simulink library "halout"  (R2021b)
settings: Solver=VariableStepAuto  StartTime=0.0  StopTime=10.0  RelTol=1e-3
undefined symbols (not defined in the file): C_TASK_5MS_S, FALSE, KHAL_CAN1FD1APS3E2E_flg, KHAL_CAN1FD1APS3TxReq_flg, KHAL_CAN1FD1VCU2E2E_flg, KHAL_CAN1FD1VCU2TxReq_flg, KHAL_CAN1FD1VCU3E2E_flg, KHAL_CAN1FD1VCU3TxReq_flg, KHAL_CAN1TxReq_flg, KHAL_CAN1VMCFCM1E2E_flg, KHAL_CAN1VMCFCM1TxReq_flg, KHAL_CAN2TxReq_flg, KHAL_CAN3FD3VCU1toNIDECTxReq_flg, KHAL_CAN3FD3VCU1TxReq_flg, KHAL_CAN3FD3VCU2E2E_flg, KHAL_CAN3FD3VCU2toNIDECE2E_flg, KHAL_CAN3FD3VCU2toNIDECTxReq_flg, KHAL_CAN3FD3VCU2TxReq_flg, KHAL_CAN3TxReq_flg, KHAL_CAN4FD4CE1000E2E_flg, KHAL_CAN4FD4CE1000TxReq_flg, KHAL_CAN4TxReq_flg, KHAL_CAN5TxReq_flg, KHAL_CAN6FD6APS3E2E_flg, KHAL_CAN6FD6APS3TxReq_flg, KHAL_CAN6FD6VCU2E2E_flg, KHAL_CAN6FD6VCU2TxReq_flg, KHAL_CAN6TxReq_flg, ONE_INT, TRUE, ZERO_INT
libraries: FVT_lib x551, simulink x244
(part 23 of 26)

== system halout/HAL_OUT/CAN4/FD4_CE100_1_0x182/RrCoolanttemp ==
  RrCoolanttemp : Inport
  Data Type Conversion : DataTypeConversion  OutDataTypeStr=uint16  RndMeth=Round
  convert_out : FVT_lib/hal/convert_out  gain=1  offset=-40
  CAN4_Rr_Coolanttemp : Outport
  wires:
  Data Type Conversion/1 -> CAN4_Rr_Coolanttemp/1
  convert_out/1 -> Data Type Conversion/1
  RrCoolanttemp/1 -> convert_out/1

== system halout/HAL_OUT/CAN4/FD4_CE100_1_0x182/sigAirIntenZon1St ==
  sigAirIntenZon1St : Inport
  Data Type Conversion : DataTypeConversion  OutDataTypeStr=uint8  RndMeth=Round
  CAN4_sigAirIntenZon1St : Outport
  wires:
  Data Type Conversion/1 -> CAN4_sigAirIntenZon1St/1
  sigAirIntenZon1St/1 -> Data Type Conversion/1

== system halout/HAL_OUT/CAN4/FD4_CE100_1_0x182/sigAirIntenZon3St ==
  sigAirIntenZon3St : Inport
  Data Type Conversion : DataTypeConversion  OutDataTypeStr=uint8  RndMeth=Round
  CAN4_sigAirIntenZon3St : Outport
  wires:
  Data Type Conversion/1 -> CAN4_sigAirIntenZon3St/1
  sigAirIntenZon3St/1 -> Data Type Conversion/1

== system halout/HAL_OUT/CAN4/FD4_CE100_1_0x182/sigAmbAirT ==
  sigAmbAirT : Inport
  Data Type Conversion : DataTypeConversion  OutDataTypeStr=uint8  RndMeth=Round
  convert_out : FVT_lib/hal/convert_out  gain=0.5  offset=-40
  CAN4_sigAmbAirT : Outport
  wires:
  Data Type Conversion/1 -> CAN4_sigAmbAirT/1
  convert_out/1 -> Data Type Conversion/1
  sigAmbAirT/1 -> convert_out/1

== system halout/HAL_OUT/CAN4/FD4_CE100_1_0x182/sigCbnAirT ==
  sigCbnAirT : Inport
  Data Type Conversion : DataTypeConversion  OutDataTypeStr=uint8  RndMeth=Round
  convert_out : FVT_lib/hal/convert_out  gain=0.5  offset=-40
  CAN4_sigCbnAirT : Outport
  wires:
  Data Type Conversion/1 -> CAN4_sigCbnAirT/1
  convert_out/1 -> Data Type Conversion/1
  sigCbnAirT/1 -> convert_out/1

== system halout/HAL_OUT/CAN4/FD4_CE100_1_0x182/sigCbnPTCPwrAct ==
  sigCbnPTCPwrAct : Inport
  Data Type Conversion : DataTypeConversion  OutDataTypeStr=uint8  RndMeth=Round
  convert_out : FVT_lib/hal/convert_out  gain=50  offset=0
  CAN4_sigCbnPTCPwrAct : Outport
  wires:
  Data Type Conversion/1 -> CAN4_sigCbnPTCPwrAct/1
  convert_out/1 -> Data Type Conversion/1
  sigCbnPTCPwrAct/1 -> convert_out/1

== system halout/HAL_OUT/CAN4/FD4_CE100_1_0x182/sigCbnSolarLeft ==
  sigCbnSolarLeft : Inport
  Data Type Conversion : DataTypeConversion  OutDataTypeStr=uint8  RndMeth=Round
  convert_out : FVT_lib/hal/convert_out  gain=5  offset=0
  CAN4_sigCbnSolarLeft : Outport
  wires:
  Data Type Conversion/1 -> CAN4_sigCbnSolarLeft/1
  convert_out/1 -> Data Type Conversion/1
  sigCbnSolarLeft/1 -> convert_out/1

== system halout/HAL_OUT/CAN4/FD4_CE100_1_0x182/sigCbnSolarRight ==
  sigCbnSolarRight : Inport
  Data Type Conversion : DataTypeConversion  OutDataTypeStr=uint8  RndMeth=Round
  convert_out : FVT_lib/hal/convert_out  gain=5  offset=0
  CAN4_sigCbnSolarRight : Outport
  wires:
  Data Type Conversion/1 -> CAN4_sigCbnSolarRight/1
  convert_out/1 -> Data Type Conversion/1
  sigCbnSolarRight/1 -> convert_out/1

== system halout/HAL_OUT/CAN4/FD4_CE100_1_0x182/sigClmtCmprPwrAct ==
  sigClmtCmprPwrAct : Inport
  Data Type Conversion : DataTypeConversion  OutDataTypeStr=uint8  RndMeth=Round
  convert_out : FVT_lib/hal/convert_out  gain=50  offset=0
  CAN4_sigClmtCmprPwrAct : Outport
  wires:
  Data Type Conversion/1 -> CAN4_sigClmtCmprPwrAct/1
  convert_out/1 -> Data Type Conversion/1
  sigClmtCmprPwrAct/1 -> convert_out/1

== system halout/HAL_OUT/CAN4/FD4_CE100_1_0x182/sigClntTHvBattOut ==
  sigClntTHvBattOut : Inport
  Data Type Conversion : DataTypeConversion  OutDataTypeStr=uint8  RndMeth=Round
  convert_out : FVT_lib/hal/convert_out  gain=0.5  offset=-40
  CAN4_sigClntTHvBattOut : Outport
  wires:
  Data Type Conversion/1 -> CAN4_sigClntTHvBattOut/1
  convert_out/1 -> Data Type Conversion/1
  sigClntTHvBattOut/1 -> convert_out/1

== system halout/HAL_OUT/CAN4/FD4_CE100_1_0x182/sigDfrstSt ==
  sigDfrstSt : Inport
  Data Type Conversion : DataTypeConversion  OutDataTypeStr=uint8  RndMeth=Round
  CAN4_sigDfrstSt : Outport
  wires:
  Data Type Conversion/1 -> CAN4_sigDfrstSt/1
  sigDfrstSt/1 -> Data Type Conversion/1

== system halout/HAL_OUT/CAN4/FD4_CE100_1_0x182/sigHvacSt ==
  sigHvacSt : Inport
  Data Type Conversion : DataTypeConversion  OutDataTypeStr=uint8  RndMeth=Round
  CAN4_sigHvacSt : Outport
  wires:
  Data Type Conversion/1 -> CAN4_sigHvacSt/1
  sigHvacSt/1 -> Data Type Conversion/1

== system halout/HAL_OUT/CAN4/FD4_CE100_1_0x182/sigRecircSt ==
  sigRecircSt : Inport
  Data Type Conversion : DataTypeConversion  OutDataTypeStr=uint8  RndMeth=Round
  CAN4_sigRecircSt : Outport
  wires:
  Data Type Conversion/1 -> CAN4_sigRecircSt/1
  sigRecircSt/1 -> Data Type Conversion/1

== system halout/HAL_OUT/CAN4/FD4_CE100_1_0x182/sigSetTempZon1St ==
  sigSetTempZon1St : Inport
  Data Type Conversion : DataTypeConversion  OutDataTypeStr=uint8  RndMeth=Round
  convert_out : FVT_lib/hal/convert_out  gain=0.5  offset=17
  CAN4_sigSetTempZon1St : Outport
  wires:
  Data Type Conversion/1 -> CAN4_sigSetTempZon1St/1
  convert_out/1 -> Data Type Conversion/1
  sigSetTempZon1St/1 -> convert_out/1

== system halout/HAL_OUT/CAN4/FD4_CE100_1_0x182/sigSetTempZon2St ==
  sigSetTempZon2St : Inport
  Data Type Conversion : DataTypeConversion  OutDataTypeStr=uint8  RndMeth=Round
  convert_out : FVT_lib/hal/convert_out  gain=0.5  offset=17
  CAN4_sigSetTempZon2St : Outport
  wires:
  Data Type Conversion/1 -> CAN4_sigSetTempZon2St/1
  convert_out/1 -> Data Type Conversion/1
  sigSetTempZon2St/1 -> convert_out/1

== system halout/HAL_OUT/CAN4/FD4_CE100_1_0x182/sigSetTempZon3St ==
  sigSetTempZon3St : Inport
  Data Type Conversion : DataTypeConversion  OutDataTypeStr=uint8  RndMeth=Round
  convert_out : FVT_lib/hal/convert_out  gain=0.5  offset=17
  CAN4_sigSetTempZon3St : Outport
  wires:
  Data Type Conversion/1 -> CAN4_sigSetTempZon3St/1
  convert_out/1 -> Data Type Conversion/1
  sigSetTempZon3St/1 -> convert_out/1

== system halout/HAL_OUT/CAN4/FD4_CE100_1_0x182/sigWindDirZon1St ==
  sigWindDirZon1St : Inport
  Data Type Conversion : DataTypeConversion  OutDataTypeStr=uint8  RndMeth=Round
  CAN4_sigWindDirZon1St : Outport
  wires:
  Data Type Conversion/1 -> CAN4_sigWindDirZon1St/1
  sigWindDirZon1St/1 -> Data Type Conversion/1

== system halout/HAL_OUT/CAN4/FD4_CE100_1_0x182/sigWindDirZon3St ==
  sigWindDirZon3St : Inport
  Data Type Conversion : DataTypeConversion  OutDataTypeStr=uint8  RndMeth=Round
  CAN4_sigWindDirZon3St : Outport
  wires:
  Data Type Conversion/1 -> CAN4_sigWindDirZon3St/1
  sigWindDirZon3St/1 -> Data Type Conversion/1

== system halout/HAL_OUT/CAN4/FD4_CE200_0_0x217/AmbLightBreath1 ==
  AmbLightBreath1 : Inport
  Data Type Conversion : DataTypeConversion  OutDataTypeStr=uint8  RndMeth=Round
  CAN4_AmbLightBreath1 : Outport
  wires:
  Data Type Conversion/1 -> CAN4_AmbLightBreath1/1
  AmbLightBreath1/1 -> Data Type Conversion/1

== system halout/HAL_OUT/CAN4/FD4_CE200_0_0x217/AmbLightBreath2 ==
  AmbLightBreath2 : Inport
  Data Type Conversion : DataTypeConversion  OutDataTypeStr=uint8  RndMeth=Round
  CAN4_AmbLightBreath2 : Outport
  wires:
  Data Type Conversion/1 -> CAN4_AmbLightBreath2/1
  AmbLightBreath2/1 -> Data Type Conversion/1

== system halout/HAL_OUT/CAN4/FD4_CE200_0_0x217/AmbLightBreath3 ==
  AmbLightBreath3 : Inport
  Data Type Conversion : DataTypeConversion  OutDataTypeStr=uint8  RndMeth=Round
  CAN4_AmbLightBreath3 : Outport
  wires:
  Data Type Conversion/1 -> CAN4_AmbLightBreath3/1
  AmbLightBreath3/1 -> Data Type Conversion/1

== system halout/HAL_OUT/CAN4/FD4_CE200_0_0x217/AmbLightBreath4 ==
  AmbLightBreath4 : Inport
  Data Type Conversion : DataTypeConversion  OutDataTypeStr=uint8  RndMeth=Round
  CAN4_AmbLightBreath4 : Outport
  wires:
  Data Type Conversion/1 -> CAN4_AmbLightBreath4/1
  AmbLightBreath4/1 -> Data Type Conversion/1

== system halout/HAL_OUT/CAN4/FD4_CE200_0_0x217/AmbLightBreath5 ==
  AmbLightBreath5 : Inport
  Data Type Conversion : DataTypeConversion  OutDataTypeStr=uint8  RndMeth=Round
  CAN4_AmbLightBreath5 : Outport
  wires:
  Data Type Conversion/1 -> CAN4_AmbLightBreath5/1
  AmbLightBreath5/1 -> Data Type Conversion/1

== system halout/HAL_OUT/CAN4/FD4_CE200_0_0x217/AmbLightBreath6 ==
  AmbLightBreath6 : Inport
  Data Type Conversion : DataTypeConversion  OutDataTypeStr=uint8  RndMeth=Round
  CAN4_AmbLightBreath6 : Outport
  wires:
  Data Type Conversion/1 -> CAN4_AmbLightBreath6/1
  AmbLightBreath6/1 -> Data Type Conversion/1

== system halout/HAL_OUT/CAN4/FD4_CE200_0_0x217/AmbLightBrightness1 ==
  AmbLightBrightness1 : Inport
  Data Type Conversion : DataTypeConversion  OutDataTypeStr=uint8  RndMeth=Round
  CAN4_AmbLightBrightness1 : Outport
  wires:
  Data Type Conversion/1 -> CAN4_AmbLightBrightness1/1
  AmbLightBrightness1/1 -> Data Type Conversion/1

== system halout/HAL_OUT/CAN4/FD4_CE200_0_0x217/AmbLightBrightness2 ==
  AmbLightBrightness2 : Inport
  Data Type Conversion : DataTypeConversion  OutDataTypeStr=uint8  RndMeth=Round
  CAN4_AmbLightBrightness2 : Outport
  wires:
  Data Type Conversion/1 -> CAN4_AmbLightBrightness2/1
  AmbLightBrightness2/1 -> Data Type Conversion/1

== system halout/HAL_OUT/CAN4/FD4_CE200_0_0x217/AmbLightBrightness3 ==
  AmbLightBrightness3 : Inport
  Data Type Conversion : DataTypeConversion  OutDataTypeStr=uint8  RndMeth=Round
  CAN4_AmbLightBrightness3 : Outport
  wires:
  Data Type Conversion/1 -> CAN4_AmbLightBrightness3/1
  AmbLightBrightness3/1 -> Data Type Conversion/1

== system halout/HAL_OUT/CAN4/FD4_CE200_0_0x217/AmbLightBrightness4 ==
  AmbLightBrightness4 : Inport
  Data Type Conversion : DataTypeConversion  OutDataTypeStr=uint8  RndMeth=Round
  CAN4_AmbLightBrightness4 : Outport
  wires:
  Data Type Conversion/1 -> CAN4_AmbLightBrightness4/1
  AmbLightBrightness4/1 -> Data Type Conversion/1

== system halout/HAL_OUT/CAN4/FD4_CE200_0_0x217/AmbLightBrightness5 ==
  AmbLightBrightness5 : Inport
  Data Type Conversion : DataTypeConversion  OutDataTypeStr=uint8  RndMeth=Round
  CAN4_AmbLightBrightness5 : Outport
  wires:
  Data Type Conversion/1 -> CAN4_AmbLightBrightness5/1
  AmbLightBrightness5/1 -> Data Type Conversion/1

== system halout/HAL_OUT/CAN4/FD4_CE200_0_0x217/AmbLightBrightness6 ==
  AmbLightBrightness6 : Inport
  Data Type Conversion : DataTypeConversion  OutDataTypeStr=uint8  RndMeth=Round
  CAN4_AmbLightBrightness6 : Outport
  wires:
  Data Type Conversion/1 -> CAN4_AmbLightBrightness6/1
  AmbLightBrightness6/1 -> Data Type Conversion/1

== system halout/HAL_OUT/CAN4/FD4_CE200_0_0x217/AmbLightColor1 ==
  AmbLightColor1 : Inport
  Data Type Conversion : DataTypeConversion  OutDataTypeStr=uint8  RndMeth=Round
  CAN4_AmbLightColor1 : Outport
  wires:
  Data Type Conversion/1 -> CAN4_AmbLightColor1/1
  AmbLightColor1/1 -> Data Type Conversion/1

== system halout/HAL_OUT/CAN4/FD4_CE200_0_0x217/AmbLightColor2 ==
  AmbLightColor2 : Inport
  Data Type Conversion : DataTypeConversion  OutDataTypeStr=uint8  RndMeth=Round
  CAN4_AmbLightColor2 : Outport
  wires:
  Data Type Conversion/1 -> CAN4_AmbLightColor2/1
  AmbLightColor2/1 -> Data Type Conversion/1

== system halout/HAL_OUT/CAN4/FD4_CE200_0_0x217/AmbLightColor3 ==
  AmbLightColor3 : Inport
  Data Type Conversion : DataTypeConversion  OutDataTypeStr=uint8  RndMeth=Round
  CAN4_AmbLightColor3 : Outport
  wires:
  Data Type Conversion/1 -> CAN4_AmbLightColor3/1
  AmbLightColor3/1 -> Data Type Conversion/1

== system halout/HAL_OUT/CAN4/FD4_CE200_0_0x217/AmbLightColor4 ==
  AmbLightColor4 : Inport
  Data Type Conversion : DataTypeConversion  OutDataTypeStr=uint8  RndMeth=Round
  CAN4_AmbLightColor4 : Outport
  wires:
  Data Type Conversion/1 -> CAN4_AmbLightColor4/1
  AmbLightColor4/1 -> Data Type Conversion/1

== system halout/HAL_OUT/CAN4/FD4_CE200_0_0x217/AmbLightColor5 ==
  AmbLightColor5 : Inport
  Data Type Conversion : DataTypeConversion  OutDataTypeStr=uint8  RndMeth=Round
  CAN4_AmbLightColor5 : Outport
  wires:
  Data Type Conversion/1 -> CAN4_AmbLightColor5/1
  AmbLightColor5/1 -> Data Type Conversion/1

== system halout/HAL_OUT/CAN4/FD4_CE200_0_0x217/AmbLightColor6 ==
  AmbLightColor6 : Inport
  Data Type Conversion : DataTypeConversion  OutDataTypeStr=uint8  RndMeth=Round
  CAN4_AmbLightColor6 : Outport
  wires:
  Data Type Conversion/1 -> CAN4_AmbLightColor6/1
  AmbLightColor6/1 -> Data Type Conversion/1

== system halout/HAL_OUT/CAN4/FD4_CE200_0_0x217/BCMBuzzerReq ==
  BCMBuzzerReq : Inport
  Data Type Conversion : DataTypeConversion  OutDataTypeStr=uint8  RndMeth=Round
  CAN4_BCM_Buzzer_Req : Outport
  wires:
  Data Type Conversion/1 -> CAN4_BCM_Buzzer_Req/1
  BCMBuzzerReq/1 -> Data Type Conversion/1

== system halout/HAL_OUT/CAN4/FD4_CE200_0_0x217/FDCBCMATCtrlCmd ==
  FDCBCMATCtrlCmd : Inport
  Data Type Conversion : DataTypeConversion  OutDataTypeStr=uint8  RndMeth=Round
  CAN4_FDC_BCM_ATCtrl_Cmd : Outport
  wires:
  Data Type Conversion/1 -> CAN4_FDC_BCM_ATCtrl_Cmd/1
  FDCBCMATCtrlCmd/1 -> Data Type Conversion/1

== system halout/HAL_OUT/CAN4/FD4_CE200_0_0x217/FDCBCMDSEATentryfsetSta ==
  FDCBCMDSEATentryfsetSta : Inport
  Data Type Conversion : DataTypeConversion  OutDataTypeStr=uint8  RndMeth=Round
  CAN4_FDC_BCM_DSEATentryfset_Sta : Outport
  wires:
  Data Type Conversion/1 -> CAN4_FDC_BCM_DSEATentryfset_Sta/1
  FDCBCMDSEATentryfsetSta/1 -> Data Type Conversion/1

== system halout/HAL_OUT/CAN4/FD4_CE200_0_0x217/FDCBCMDimSw ==
  FDCBCMDimSw : Inport
  Data Type Conversion : DataTypeConversion  OutDataTypeStr=uint8  RndMeth=Round
  CAN4_FDC_BCM_DimSw : Outport
  wires:
  Data Type Conversion/1 -> CAN4_FDC_BCM_DimSw/1
  FDCBCMDimSw/1 -> Data Type Conversion/1

== system halout/HAL_OUT/CAN4/FD4_CE200_0_0x217/FDCBCMDrHandleLampCmd ==
  FDCBCMDrHandleLampCmd : Inport
  Data Type Conversion : DataTypeConversion  OutDataTypeStr=uint8  RndMeth=Round
  CAN4_FDC_BCM_DrHandleLamp_Cmd : Outport
  wires:
  Data Type Conversion/1 -> CAN4_FDC_BCM_DrHandleLamp_Cmd/1
  FDCBCMDrHandleLampCmd/1 -> Data Type Conversion/1

== system halout/HAL_OUT/CAN4/FD4_CE200_0_0x217/FDCBCMDrRWdwReqAPSta ==
  FDCBCMDrRWdwReqAPSta : Inport
  Data Type Conversion : DataTypeConversion  OutDataTypeStr=uint8  RndMeth=Round
  CAN4_FDC_BCM_DrRWdwReqAP_Sta : Outport
  wires:
  Data Type Conversion/1 -> CAN4_FDC_BCM_DrRWdwReqAP_Sta/1
  FDCBCMDrRWdwReqAPSta/1 -> Data Type Conversion/1

== system halout/HAL_OUT/CAN4/FD4_CE200_0_0x217/FDCBCMDrvWdwReqAPSta ==
  FDCBCMDrvWdwReqAPSta : Inport
  Data Type Conversion : DataTypeConversion  OutDataTypeStr=uint8  RndMeth=Round
  CAN4_FDC_BCM_DrvWdwReqAP_Sta : Outport
  wires:
  Data Type Conversion/1 -> CAN4_FDC_BCM_DrvWdwReqAP_Sta/1
  FDCBCMDrvWdwReqAPSta/1 -> Data Type Conversion/1

== system halout/HAL_OUT/CAN4/FD4_CE200_0_0x217/FDCBCMFWasSwSta ==
  FDCBCMFWasSwSta : Inport
  Data Type Conversion : DataTypeConversion  OutDataTypeStr=uint8  RndMeth=Round
  CAN4_FDC_BCM_FWasSw_Sta : Outport
  wires:
  Data Type Conversion/1 -> CAN4_FDC_BCM_FWasSw_Sta/1
  FDCBCMFWasSwSta/1 -> Data Type Conversion/1

== system halout/HAL_OUT/CAN4/FD4_CE200_0_0x217/FDCBCMFWipSwSta ==
  FDCBCMFWipSwSta : Inport
  Data Type Conversion : DataTypeConversion  OutDataTypeStr=uint8  RndMeth=Round
  CAN4_FDC_BCM_FWipSw_Sta : Outport
  wires:
  Data Type Conversion/1 -> CAN4_FDC_BCM_FWipSw_Sta/1
  FDCBCMFWipSwSta/1 -> Data Type Conversion/1

== system halout/HAL_OUT/CAN4/FD4_CE200_0_0x217/FDCBCMHBeamADBCmd ==
  FDCBCMHBeamADBCmd : Inport
  Data Type Conversion : DataTypeConversion  OutDataTypeStr=uint8  RndMeth=Round
  CAN4_FDC_BCM_HBeamADB_Cmd : Outport
  wires:
  Data Type Conversion/1 -> CAN4_FDC_BCM_HBeamADB_Cmd/1
  FDCBCMHBeamADBCmd/1 -> Data Type Conversion/1

== system halout/HAL_OUT/CAN4/FD4_CE200_0_0x217/FDCBCMHandleControlCmd ==
  FDCBCMHandleControlCmd : Inport
  Data Type Conversion : DataTypeConversion  OutDataTypeStr=uint8  RndMeth=Round
  CAN4_FDC_BCM_HandleControl_Cmd : Outport
  wires:
  Data Type Conversion/1 -> CAN4_FDC_BCM_HandleControl_Cmd/1
  FDCBCMHandleControlCmd/1 -> Data Type Conversion/1

== system halout/HAL_OUT/CAN4/FD4_CE200_0_0x217/FDCBCMHazardINDCmd ==
  FDCBCMHazardINDCmd : Inport
  Data Type Conversion : DataTypeConversion  OutDataTypeStr=uint8  RndMeth=Round
  CAN4_FDC_BCM_HazardIND_Cmd : Outport
  wires:
  Data Type Conversion/1 -> CAN4_FDC_BCM_HazardIND_Cmd/1
  FDCBCMHazardINDCmd/1 -> Data Type Conversion/1

== system halout/HAL_OUT/CAN4/FD4_CE200_0_0x217/FDCBCMHoodRelCmd ==
  FDCBCMHoodRelCmd : Inport
  Data Type Conversion : DataTypeConversion  OutDataTypeStr=uint8  RndMeth=Round
  CAN4_FDC_BCM_HoodRel_Cmd : Outport
  wires:
  Data Type Conversion/1 -> CAN4_FDC_BCM_HoodRel_Cmd/1
  FDCBCMHoodRelCmd/1 -> Data Type Conversion/1

== system halout/HAL_OUT/CAN4/FD4_CE200_0_0x217/FDCBCMLPSDCtrlCmd ==
  FDCBCMLPSDCtrlCmd : Inport
  Data Type Conversion : DataTypeConversion  OutDataTypeStr=uint8  RndMeth=Round
  CAN4_FDC_BCM_LPSDCtrl_Cmd : Outport
  wires:
  Data Type Conversion/1 -> CAN4_FDC_BCM_LPSDCtrl_Cmd/1
  FDCBCMLPSDCtrlCmd/1 -> Data Type Conversion/1

== system halout/HAL_OUT/CAN4/FD4_CE200_0_0x217/FDCBCMLockAlarmCmd ==
  FDCBCMLockAlarmCmd : Inport
  Data Type Conversion : DataTypeConversion  OutDataTypeStr=uint8  RndMeth=Round
  CAN4_FDC_BCM_LockAlarm_Cmd : Outport
  wires:
  Data Type Conversion/1 -> CAN4_FDC_BCM_LockAlarm_Cmd/1
  FDCBCMLockAlarmCmd/1 -> Data Type Conversion/1

== system halout/HAL_OUT/CAN4/FD4_CE200_0_0x217/FDCBCMOtHandleLampCmd ==
  FDCBCMOtHandleLampCmd : Inport
  Data Type Conversion : DataTypeConversion  OutDataTypeStr=uint8  RndMeth=Round
  CAN4_FDC_BCM_OtHandleLamp_Cmd : Outport
  wires:
  Data Type Conversion/1 -> CAN4_FDC_BCM_OtHandleLamp_Cmd/1
  FDCBCMOtHandleLampCmd/1 -> Data Type Conversion/1

== system halout/HAL_OUT/CAN4/FD4_CE200_0_0x217/FDCBCMOutModeCmd ==
  FDCBCMOutModeCmd : Inport
  Data Type Conversion : DataTypeConversion  OutDataTypeStr=uint8  RndMeth=Round
  CAN4_FDC_BCM_OutMode_Cmd : Outport
  wires:
  Data Type Conversion/1 -> CAN4_FDC_BCM_OutMode_Cmd/1
  FDCBCMOutModeCmd/1 -> Data Type Conversion/1

== system halout/HAL_OUT/CAN4/FD4_CE200_0_0x217/FDCBCMPTGOpenHeightSta ==
  FDCBCMPTGOpenHeightSta : Inport
  Data Type Conversion : DataTypeConversion  OutDataTypeStr=uint8  RndMeth=Round
  CAN4_FDC_BCM_PTGOpenHeight_Sta : Outport
  wires:
  Data Type Conversion/1 -> CAN4_FDC_BCM_PTGOpenHeight_Sta/1
  FDCBCMPTGOpenHeightSta/1 -> Data Type Conversion/1

== system halout/HAL_OUT/CAN4/FD4_CE200_0_0x217/FDCBCMPasWdwReqAPSta ==
  FDCBCMPasWdwReqAPSta : Inport
  Data Type Conversion : DataTypeConversion  OutDataTypeStr=uint8  RndMeth=Round
  CAN4_FDC_BCM_PasWdwReqAP_Sta : Outport
  wires:
  Data Type Conversion/1 -> CAN4_FDC_BCM_PasWdwReqAP_Sta/1
  FDCBCMPasWdwReqAPSta/1 -> Data Type Conversion/1

== system halout/HAL_OUT/CAN4/FD4_CE200_0_0x217/FDCBCMPassSWSta ==
  FDCBCMPassSWSta : Inport
  Data Type Conversion : DataTypeConversion  OutDataTypeStr=uint8  RndMeth=Round
  CAN4_FDC_BCM_PassSW_Sta : Outport
  wires:
  Data Type Conversion/1 -> CAN4_FDC_BCM_PassSW_Sta/1
  FDCBCMPassSWSta/1 -> Data Type Conversion/1

== system halout/HAL_OUT/CAN4/FD4_CE200_0_0x217/FDCBCMPsRWdwReqAPSta ==
  FDCBCMPsRWdwReqAPSta : Inport
  Data Type Conversion : DataTypeConversion  OutDataTypeStr=uint8  RndMeth=Round
  CAN4_FDC_BCM_PsRWdwReqAP_Sta : Outport
  wires:
  Data Type Conversion/1 -> CAN4_FDC_BCM_PsRWdwReqAP_Sta/1
  FDCBCMPsRWdwReqAPSta/1 -> Data Type Conversion/1

== system halout/HAL_OUT/CAN4/FD4_CE200_0_0x217/FDCBCMRPSDCtrlCmd ==
  FDCBCMRPSDCtrlCmd : Inport
  Data Type Conversion : DataTypeConversion  OutDataTypeStr=uint8  RndMeth=Round
  CAN4_FDC_BCM_RPSDCtrl_Cmd : Outport
  wires:
  Data Type Conversion/1 -> CAN4_FDC_BCM_RPSDCtrl_Cmd/1
  FDCBCMRPSDCtrlCmd/1 -> Data Type Conversion/1

== system halout/HAL_OUT/CAN4/FD4_CE200_0_0x217/FDCBCMSettingUpdateReqCmd ==
  FDCBCMSettingUpdateReqCmd : Inport
  Data Type Conversion : DataTypeConversion  OutDataTypeStr=uint8  RndMeth=Round
  CAN4_FDC_BCM_SettingUpdateReq_Cmd : Outport
  wires:
  Data Type Conversion/1 -> CAN4_FDC_BCM_SettingUpdateReq_Cmd/1
  FDCBCMSettingUpdateReqCmd/1 -> Data Type Conversion/1

== system halout/HAL_OUT/CAN4/FD4_CE200_0_0x217/FDCBCMTurnSwSta ==
  FDCBCMTurnSwSta : Inport
  Data Type Conversion : DataTypeConversion  OutDataTypeStr=uint8  RndMeth=Round
  CAN4_FDC_BCM_TurnSw_Sta : Outport
  wires:
  Data Type Conversion/1 -> CAN4_FDC_BCM_TurnSw_Sta/1
  FDCBCMTurnSwSta/1 -> Data Type Conversion/1

== system halout/HAL_OUT/CAN4/FD4_CE200_0_0x217/FDCBCMTurnSwTSetStaSta ==
  FDCBCMTurnSwTSetStaSta : Inport
  Data Type Conversion : DataTypeConversion  OutDataTypeStr=uint8  RndMeth=Round
  CAN4_FDC_BCM_TurnSwTSetSta_Sta : Outport
  wires:
  Data Type Conversion/1 -> CAN4_FDC_BCM_TurnSwTSetSta_Sta/1
  FDCBCMTurnSwTSetStaSta/1 -> Data Type Conversion/1

== system halout/HAL_OUT/CAN4/FD4_CE200_0_0x217/FDCBCMUserHeightSetSta ==
  FDCBCMUserHeightSetSta : Inport
  Data Type Conversion : DataTypeConversion  OutDataTypeStr=uint16  RndMeth=Round
  CAN4_FDC_BCM_UserHeightSet_Sta : Outport
  wires:
  Data Type Conversion/1 -> CAN4_FDC_BCM_UserHeightSet_Sta/1
  FDCBCMUserHeightSetSta/1 -> Data Type Conversion/1

== system halout/HAL_OUT/CAN4/FD4_CE200_0_0x217/FDCBCMUserNowSta ==
  FDCBCMUserNowSta : Inport
  Data Type Conversion : DataTypeConversion  OutDataTypeStr=uint8  RndMeth=Round
  CAN4_FDC_BCM_UserNow_Sta : Outport
  wires:
  Data Type Conversion/1 -> CAN4_FDC_BCM_UserNow_Sta/1
  FDCBCMUserNowSta/1 -> Data Type Conversion/1

== system halout/HAL_OUT/CAN4/FD4_CE200_0_0x217/FDCDKCCommandToBCMCmd ==
  FDCDKCCommandToBCMCmd : Inport
  Data Type Conversion : DataTypeConversion  OutDataTypeStr=uint8  RndMeth=Round
  CAN4_FDC_DKC_CommandToBCM_Cmd : Outport
  wires:
  Data Type Conversion/1 -> CAN4_FDC_DKC_CommandToBCM_Cmd/1
  FDCDKCCommandToBCMCmd/1 -> Data Type Conversion/1

== system halout/HAL_OUT/CAN4/FD4_CE200_0_0x217/FDCDKCDKeyAreaPESta ==
  FDCDKCDKeyAreaPESta : Inport
  Data Type Conversion : DataTypeConversion  OutDataTypeStr=uint8  RndMeth=Round
  CAN4_FDC_DKC_DKeyAreaPE_Sta : Outport
  wires:
  Data Type Conversion/1 -> CAN4_FDC_DKC_DKeyAreaPE_Sta/1
  FDCDKCDKeyAreaPESta/1 -> Data Type Conversion/1

== system halout/HAL_OUT/CAN4/FD4_CE200_0_0x217/FDCDKCSPTGDetCmd ==
  FDCDKCSPTGDetCmd : Inport
  Data Type Conversion : DataTypeConversion  OutDataTypeStr=uint8  RndMeth=Round
  CAN4_FDC_DKC_SPTGDet_Cmd : Outport
  wires:
  Data Type Conversion/1 -> CAN4_FDC_DKC_SPTGDet_Cmd/1
  FDCDKCSPTGDetCmd/1 -> Data Type Conversion/1

== system halout/HAL_OUT/CAN4/FD4_CE200_0_0x217/FDCDKCSPTGOpenCmd ==
  FDCDKCSPTGOpenCmd : Inport
  Data Type Conversion : DataTypeConversion  OutDataTypeStr=uint8  RndMeth=Round
  CAN4_FDC_DKC_SPTGOpen_Cmd : Outport
  wires:
  Data Type Conversion/1 -> CAN4_FDC_DKC_SPTGOpen_Cmd/1
  FDCDKCSPTGOpenCmd/1 -> Data Type Conversion/1

== system halout/HAL_OUT/CAN4/FD4_CE200_0_0x217/FDCFGSAirIntCmd ==
  FDCFGSAirIntCmd : Inport
  Data Type Conversion : DataTypeConversion  OutDataTypeStr=uint8  RndMeth=Round
  CAN4_FDC_FGS_AirInt_Cmd : Outport
  wires:
  Data Type Conversion/1 -> CAN4_FDC_FGS_AirInt_Cmd/1
  FDCFGSAirIntCmd/1 -> Data Type Conversion/1

== system halout/HAL_OUT/CAN4/FD4_CE200_0_0x217/FDCFGSFGSChCmd ==
  FDCFGSFGSChCmd : Inport
  Data Type Conversion : DataTypeConversion  OutDataTypeStr=uint8  RndMeth=Round
  CAN4_FDC_FGS_FGSCh_Cmd : Outport
  wires:
  Data Type Conversion/1 -> CAN4_FDC_FGS_FGSCh_Cmd/1
  FDCFGSFGSChCmd/1 -> Data Type Conversion/1

== system halout/HAL_OUT/CAN4/FD4_CE200_0_0x217/FDCFGSFuncStaCmd ==
  FDCFGSFuncStaCmd : Inport
  Data Type Conversion : DataTypeConversion  OutDataTypeStr=uint8  RndMeth=Round
  CAN4_FDC_FGS_FuncSta_Cmd : Outport
  wires:
  Data Type Conversion/1 -> CAN4_FDC_FGS_FuncSta_Cmd/1
  FDCFGSFuncStaCmd/1 -> Data Type Conversion/1

== system halout/HAL_OUT/CAN4/FD4_CE200_0_0x217/FDCFGSIONCmd ==
  FDCFGSIONCmd : Inport
  Data Type Conversion : DataTypeConversion  OutDataTypeStr=uint8  RndMeth=Round
  CAN4_FDC_FGS_ION_Cmd : Outport
  wires:
  Data Type Conversion/1 -> CAN4_FDC_FGS_ION_Cmd/1
  FDCFGSIONCmd/1 -> Data Type Conversion/1

== system halout/HAL_OUT/CAN4/FD4_CE200_0_0x217/FDCTHCMACTInitialCmd ==
  FDCTHCMACTInitialCmd : Inport
  Data Type Conversion : DataTypeConversion  OutDataTypeStr=uint8  RndMeth=Round
  CAN4_FDC_THCM_ACTInitial_Cmd : Outport
  wires:
  Data Type Conversion/1 -> CAN4_FDC_THCM_ACTInitial_Cmd/1
  FDCTHCMACTInitialCmd/1 -> Data Type Conversion/1

== system halout/HAL_OUT/CAN4/FD4_CE200_0_0x217/FDCTHCMAirIntZ3Sta ==
  FDCTHCMAirIntZ3Sta : Inport
  Data Type Conversion : DataTypeConversion  OutDataTypeStr=uint8  RndMeth=Round
  CAN4_FDC_THCM_AirIntZ3_Sta : Outport
  wires:
  Data Type Conversion/1 -> CAN4_FDC_THCM_AirIntZ3_Sta/1
  FDCTHCMAirIntZ3Sta/1 -> Data Type Conversion/1

== system halout/HAL_OUT/CAN4/FD4_CE200_0_0x217/FDCV2LHVPOBklgtingCmd ==
  FDCV2LHVPOBklgtingCmd : Inport
  Data Type Conversion : DataTypeConversion  OutDataTypeStr=uint8  RndMeth=Round
  CAN4_FDC_V2L_HVPOBklgting_Cmd : Outport
  wires:
  Data Type Conversion/1 -> CAN4_FDC_V2L_HVPOBklgting_Cmd/1
  FDCV2LHVPOBklgtingCmd/1 -> Data Type Conversion/1

== system halout/HAL_OUT/CAN4/FD4_CE200_0_0x217/FDCV2LHVPOLEDStsCmd ==
  FDCV2LHVPOLEDStsCmd : Inport
  Data Type Conversion : DataTypeConversion  OutDataTypeStr=uint8  RndMeth=Round
  CAN4_FDC_V2L_HVPOLEDSts_Cmd : Outport
  wires:
  Data Type Conversion/1 -> CAN4_FDC_V2L_HVPOLEDSts_Cmd/1
  FDCV2LHVPOLEDStsCmd/1 -> Data Type Conversion/1

== system halout/HAL_OUT/CAN4/FD4_CE200_0_0x217/WelcomeLight ==
  WelcomeLight : Inport
  Data Type Conversion : DataTypeConversion  OutDataTypeStr=uint8  RndMeth=Round
  CAN4_WelcomeLight : Outport
  wires:
  Data Type Conversion/1 -> CAN4_WelcomeLight/1
  WelcomeLight/1 -> Data Type Conversion/1

== system halout/HAL_OUT/CAN4/GW4_CE100_0_0x253/FDCBCMDrRWdwCtrlCmd ==
  FDCBCMDrRWdwCtrlCmd : Inport
  Data Type Conversion : DataTypeConversion  OutDataTypeStr=uint8  RndMeth=Round
  CAN4_FDC_BCM_DrRWdwCtrl_Cmd : Outport
  wires:
  Data Type Conversion/1 -> CAN4_FDC_BCM_DrRWdwCtrl_Cmd/1
  FDCBCMDrRWdwCtrlCmd/1 -> Data Type Conversion/1

== system halout/HAL_OUT/CAN4/GW4_CE100_0_0x253/FDCBCMDrvWdwCtrlCmd ==
  FDCBCMDrvWdwCtrlCmd : Inport
  Data Type Conversion : DataTypeConversion  OutDataTypeStr=uint8  RndMeth=Round
  CAN4_FDC_BCM_DrvWdwCtrl_Cmd : Outport
  wires:
  Data Type Conversion/1 -> CAN4_FDC_BCM_DrvWdwCtrl_Cmd/1
  FDCBCMDrvWdwCtrlCmd/1 -> Data Type Conversion/1

== system halout/HAL_OUT/CAN4/GW4_CE100_0_0x253/FDCBCMPasWdwCtrlCmd ==
  FDCBCMPasWdwCtrlCmd : Inport
  Data Type Conversion : DataTypeConversion  OutDataTypeStr=uint8  RndMeth=Round
  CAN4_FDC_BCM_PasWdwCtrl_Cmd : Outport
  wires:
  Data Type Conversion/1 -> CAN4_FDC_BCM_PasWdwCtrl_Cmd/1
  FDCBCMPasWdwCtrlCmd/1 -> Data Type Conversion/1

== system halout/HAL_OUT/CAN4/GW4_CE100_0_0x253/FDCBCMPsRWdwCtrlCmd ==
  FDCBCMPsRWdwCtrlCmd : Inport
  Data Type Conversion : DataTypeConversion  OutDataTypeStr=uint8  RndMeth=Round
  CAN4_FDC_BCM_PsRWdwCtrl_Cmd : Outport
  wires:
  Data Type Conversion/1 -> CAN4_FDC_BCM_PsRWdwCtrl_Cmd/1
  FDCBCMPsRWdwCtrlCmd/1 -> Data Type Conversion/1

== system halout/HAL_OUT/CAN4/GW4_CE100_0_0x253/FDCBCMSenstivityPosnCmd ==
  FDCBCMSenstivityPosnCmd : Inport
  Data Type Conversion : DataTypeConversion  OutDataTypeStr=uint8  RndMeth=Round
  CAN4_FDC_BCM_SenstivityPosn_Cmd : Outport
  wires:
  Data Type Conversion/1 -> CAN4_FDC_BCM_SenstivityPosn_Cmd/1
  FDCBCMSenstivityPosnCmd/1 -> Data Type Conversion/1

== system halout/HAL_OUT/CAN4/GW4_CE100_0_0x253/FDCPTGinnerSW2 ==
  FDCPTGinnerSW2 : Inport
  Data Type Conversion : DataTypeConversion  OutDataTypeStr=uint8  RndMeth=Round
  CAN4_FDC_PTG_inner_SW_2 : Outport
  wires:
  Data Type Conversion/1 -> CAN4_FDC_PTG_inner_SW_2/1
  FDCPTGinnerSW2/1 -> Data Type Conversion/1

== system halout/HAL_OUT/CAN5/FD5_CE100_0_0x118/AllDoorSW ==
  AllDoorSW : Inport
  Data Type Conversion : DataTypeConversion  OutDataTypeStr=uint8  RndMeth=Round
  CAN5_AllDoorSW : Outport
  wires:
  Data Type Conversion/1 -> CAN5_AllDoorSW/1
  AllDoorSW/1 -> Data Type Conversion/1

== system halout/HAL_OUT/CAN5/FD5_CE100_0_0x118/AntitheftSta ==
  AntitheftSta : Inport
  Data Type Conversion : DataTypeConversion  OutDataTypeStr=uint8  RndMeth=Round
  CAN5_AntitheftSta : Outport
  wires:
  Data Type Conversion/1 -> CAN5_AntitheftSta/1
  AntitheftSta/1 -> Data Type Conversion/1

== system halout/HAL_OUT/CAN5/FD5_CE100_0_0x118/BCMDoorLockSta ==
  BCMDoorLockSta : Inport
  Data Type Conversion : DataTypeConversion  OutDataTypeStr=uint8  RndMeth=Round
  CAN5_BCM_DoorLock_Sta : Outport
  wires:
  Data Type Conversion/1 -> CAN5_BCM_DoorLock_Sta/1
  BCMDoorLockSta/1 -> Data Type Conversion/1

== system halout/HAL_OUT/CAN5/FD5_CE100_0_0x118/CCUACLampSts ==
  CCUACLampSts : Inport
  Data Type Conversion : DataTypeConversion  OutDataTypeStr=uint8  RndMeth=Round
  CAN5_CCU_ACLampSts : Outport
  wires:
  Data Type Conversion/1 -> CAN5_CCU_ACLampSts/1
  CCUACLampSts/1 -> Data Type Conversion/1

== system halout/HAL_OUT/CAN5/FD5_CE100_0_0x118/CCUCbnPreACWkSts ==
  CCUCbnPreACWkSts : Inport
  Data Type Conversion : DataTypeConversion  OutDataTypeStr=uint8  RndMeth=Round
  CAN5_CCU_CbnPreACWkSts : Outport
  wires:
  Data Type Conversion/1 -> CAN5_CCU_CbnPreACWkSts/1
  CCUCbnPreACWkSts/1 -> Data Type Conversion/1

== system halout/HAL_OUT/CAN5/FD5_CE100_0_0x118/CCUCbnPreEstimdTi ==
  CCUCbnPreEstimdTi : Inport
  Data Type Conversion : DataTypeConversion  OutDataTypeStr=uint8  RndMeth=Round
  CAN5_CCU_CbnPreEstimdTi : Outport
  wires:
  Data Type Conversion/1 -> CAN5_CCU_CbnPreEstimdTi/1
  CCUCbnPreEstimdTi/1 -> Data Type Conversion/1

== system halout/HAL_OUT/CAN5/FD5_CE100_0_0x118/CCUCbnPreSts ==
  CCUCbnPreSts : Inport
  Data Type Conversion : DataTypeConversion  OutDataTypeStr=uint8  RndMeth=Round
  CAN5_CCU_CbnPreSts : Outport
  wires:
  Data Type Conversion/1 -> CAN5_CCU_CbnPreSts/1
  CCUCbnPreSts/1 -> Data Type Conversion/1

== system halout/HAL_OUT/CAN5/FD5_CE100_0_0x118/FDTBOXDTCDataErr ==
  FDTBOXDTCDataErr : Inport
  Data Type Conversion : DataTypeConversion  OutDataTypeStr=uint8  RndMeth=Round
  CAN5_FD_TBOX_DTCData_Err : Outport
  wires:
  Data Type Conversion/1 -> CAN5_FD_TBOX_DTCData_Err/1
  FDTBOXDTCDataErr/1 -> Data Type Conversion/1

== system halout/HAL_OUT/CAN5/FD5_CE100_0_0x118/FDTBOXDTCDataSta ==
  FDTBOXDTCDataSta : Inport
  Data Type Conversion : DataTypeConversion  OutDataTypeStr=uint8  RndMeth=Round
  CAN5_FD_TBOX_DTCData_Sta : Outport
  wires:
  Data Type Conversion/1 -> CAN5_FD_TBOX_DTCData_Sta/1
  FDTBOXDTCDataSta/1 -> Data Type Conversion/1

== system halout/HAL_OUT/CAN5/FD5_CE100_0_0x118/FDTBOXVehDataErr ==
  FDTBOXVehDataErr : Inport
  Data Type Conversion : DataTypeConversion  OutDataTypeStr=uint8  RndMeth=Round
  CAN5_FD_TBOX_VehData_Err : Outport
  wires:
  Data Type Conversion/1 -> CAN5_FD_TBOX_VehData_Err/1
  FDTBOXVehDataErr/1 -> Data Type Conversion/1

== system halout/HAL_OUT/CAN5/FD5_CE100_0_0x118/FDTBOXVehDataSta ==
  FDTBOXVehDataSta : Inport
  Data Type Conversion : DataTypeConversion  OutDataTypeStr=uint8  RndMeth=Round
  CAN5_FD_TBOX_VehData_Sta : Outport
  wires:
  Data Type Conversion/1 -> CAN5_FD_TBOX_VehData_Sta/1
  FDTBOXVehDataSta/1 -> Data Type Conversion/1

== system halout/HAL_OUT/CAN5/FD5_CE100_0_0x118/HoodSW ==
  HoodSW : Inport
  Data Type Conversion : DataTypeConversion  OutDataTypeStr=uint8  RndMeth=Round
  CAN5_HoodSW : Outport
  wires:
  Data Type Conversion/1 -> CAN5_HoodSW/1
  HoodSW/1 -> Data Type Conversion/1

== system halout/HAL_OUT/CAN5/FD5_CE100_0_0x118/LowSOCWarn ==
  LowSOCWarn : Inport
  Data Type Conversion : DataTypeConversion  OutDataTypeStr=uint8  RndMeth=Round
  CAN5_LowSOCWarn : Outport
  wires:
  Data Type Conversion/1 -> CAN5_LowSOCWarn/1
  LowSOCWarn/1 -> Data Type Conversion/1

== system halout/HAL_OUT/CAN5/FD5_CE100_0_0x118/PwrSta ==
  PwrSta : Inport
  Data Type Conversion : DataTypeConversion  OutDataTypeStr=uint8  RndMeth=Round
  CAN5_PwrSta : Outport
  wires:
  Data Type Conversion/1 -> CAN5_PwrSta/1
  PwrSta/1 -> Data Type Conversion/1

== system halout/HAL_OUT/CAN5/FD5_CE100_0_0x118/ReVehThdChkSta ==
  ReVehThdChkSta : Inport
  Data Type Conversion : DataTypeConversion  OutDataTypeStr=uint8  RndMeth=Round
  CAN5_Re_VehThdChkSta : Outport
  wires:
  Data Type Conversion/1 -> CAN5_Re_VehThdChkSta/1
  ReVehThdChkSta/1 -> Data Type Conversion/1

== system halout/HAL_OUT/CAN5/FD5_CE100_0_0x118/ShiftGearPosn ==
  ShiftGearPosn : Inport
  Data Type Conversion : DataTypeConversion  OutDataTypeStr=uint8  RndMeth=Round
  CAN5_ShiftGearPosn : Outport
  wires:
  Data Type Conversion/1 -> CAN5_ShiftGearPosn/1
  ShiftGearPosn/1 -> Data Type Conversion/1

== system halout/HAL_OUT/CAN5/FD5_CE100_0_0x118/TCountSta ==
  TCountSta : Inport
  Data Type Conversion : DataTypeConversion  OutDataTypeStr=uint8  RndMeth=Round
  CAN5_TCountSta : Outport
  wires:
  Data Type Conversion/1 -> CAN5_TCountSta/1
  TCountSta/1 -> Data Type Conversion/1

== system halout/HAL_OUT/CAN5/FD5_CE100_0_0x118/TailgateRemote ==
  TailgateRemote : Inport
  Data Type Conversion : DataTypeConversion  OutDataTypeStr=uint8  RndMeth=Round
  CAN5_TailgateRemote : Outport
  wires:
  Data Type Conversion/1 -> CAN5_TailgateRemote/1
  TailgateRemote/1 -> Data Type Conversion/1

== system halout/HAL_OUT/CAN5/FD5_CE100_0_0x118/TailgateSW ==
  TailgateSW : Inport
  Data Type Conversion : DataTypeConversion  OutDataTypeStr=uint8  RndMeth=Round
  CAN5_Tailgate_SW : Outport
  wires:
  Data Type Conversion/1 -> CAN5_Tailgate_SW/1
  TailgateSW/1 -> Data Type Conversion/1

== system halout/HAL_OUT/CAN5/FD5_CE100_0_0x118/VehMalfunLevel ==
  VehMalfunLevel : Inport
  Data Type Conversion : DataTypeConversion  OutDataTypeStr=uint8  RndMeth=Round
  CAN5_VehMalfunLevel : Outport
  wires:
  Data Type Conversion/1 -> CAN5_VehMalfunLevel/1
  VehMalfunLevel/1 -> Data Type Conversion/1

== system halout/HAL_OUT/CAN5/FD5_Debug1_0x4D0/ID1ALTU ==
  ID1ALTU : Inport
  Data Type Conversion : DataTypeConversion  OutDataTypeStr=uint32  RndMeth=Round
  CAN5_ID1_ALTU : Outport
  wires:
  Data Type Conversion/1 -> CAN5_ID1_ALTU/1
  ID1ALTU/1 -> Data Type Conversion/1

== system halout/HAL_OUT/CAN5/FD5_Debug1_0x4D0/ID1LocALTU ==
  ID1LocALTU : Inport
  Data Type Conversion : DataTypeConversion  OutDataTypeStr=uint8  RndMeth=Round
  CAN5_ID1_Loc_ALTU : Outport
  wires:
  Data Type Conversion/1 -> CAN5_ID1_Loc_ALTU/1
  ID1LocALTU/1 -> Data Type Conversion/1

== system halout/HAL_OUT/CAN5/FD5_Debug1_0x4D0/ID1messageALTU ==
  ID1messageALTU : Inport
  Data Type Conversion : DataTypeConversion  OutDataTypeStr=uint8  RndMeth=Round
  CAN5_ID1_message_ALTU : Outport
  wires:
  Data Type Conversion/1 -> CAN5_ID1_message_ALTU/1
  ID1messageALTU/1 -> Data Type Conversion/1

== system halout/HAL_OUT/CAN5/FD5_Debug1_0x4D0/ID2ALTU ==
  ID2ALTU : Inport
  Data Type Conversion : DataTypeConversion  OutDataTypeStr=uint32  RndMeth=Round
  CAN5_ID2_ALTU : Outport
  wires:
  Data Type Conversion/1 -> CAN5_ID2_ALTU/1
  ID2ALTU/1 -> Data Type Conversion/1

== system halout/HAL_OUT/CAN5/FD5_Debug1_0x4D0/ID2LocALTU ==
  ID2LocALTU : Inport
  Data Type Conversion : DataTypeConversion  OutDataTypeStr=uint8  RndMeth=Round
  CAN5_ID2_Loc_ALTU : Outport
  wires:
  Data Type Conversion/1 -> CAN5_ID2_Loc_ALTU/1
  ID2LocALTU/1 -> Data Type Conversion/1

== system halout/HAL_OUT/CAN5/FD5_Debug1_0x4D0/ID2messageALTU ==
  ID2messageALTU : Inport
  Data Type Conversion : DataTypeConversion  OutDataTypeStr=uint8  RndMeth=Round
  CAN5_ID2_message_ALTU : Outport
  wires:
  Data Type Conversion/1 -> CAN5_ID2_message_ALTU/1
  ID2messageALTU/1 -> Data Type Conversion/1

== system halout/HAL_OUT/CAN5/FD5_Debug1_0x4D0/ID3ALTU ==
  ID3ALTU : Inport
  Data Type Conversion : DataTypeConversion  OutDataTypeStr=uint32  RndMeth=Round
  CAN5_ID3_ALTU : Outport
  wires:
  Data Type Conversion/1 -> CAN5_ID3_ALTU/1
  ID3ALTU/1 -> Data Type Conversion/1

== system halout/HAL_OUT/CAN5/FD5_Debug1_0x4D0/ID3LocALTU ==
  ID3LocALTU : Inport
  Data Type Conversion : DataTypeConversion  OutDataTypeStr=uint8  RndMeth=Round
  CAN5_ID3_Loc_ALTU : Outport
  wires:
  Data Type Conversion/1 -> CAN5_ID3_Loc_ALTU/1
  ID3LocALTU/1 -> Data Type Conversion/1

== system halout/HAL_OUT/CAN5/FD5_Debug1_0x4D0/ID3messageALTU ==
  ID3messageALTU : Inport
  Data Type Conversion : DataTypeConversion  OutDataTypeStr=uint8  RndMeth=Round
  CAN5_ID3_message_ALTU : Outport
  wires:
  Data Type Conversion/1 -> CAN5_ID3_message_ALTU/1
  ID3messageALTU/1 -> Data Type Conversion/1

== system halout/HAL_OUT/CAN5/FD5_Debug1_0x4D0/ID4ALTU ==
  ID4ALTU : Inport
  Data Type Conversion : DataTypeConversion  OutDataTypeStr=uint32  RndMeth=Round
  CAN5_ID4_ALTU : Outport
  wires:
  Data Type Conversion/1 -> CAN5_ID4_ALTU/1
  ID4ALTU/1 -> Data Type Conversion/1

== system halout/HAL_OUT/CAN5/FD5_Debug1_0x4D0/ID4LocALTU ==
  ID4LocALTU : Inport
  Data Type Conversion : DataTypeConversion  OutDataTypeStr=uint8  RndMeth=Round
  CAN5_ID4_Loc_ALTU : Outport
  wires:
  Data Type Conversion/1 -> CAN5_ID4_Loc_ALTU/1
  ID4LocALTU/1 -> Data Type Conversion/1

== system halout/HAL_OUT/CAN5/FD5_Debug1_0x4D0/ID4messageALTU ==
  ID4messageALTU : Inport
  Data Type Conversion : DataTypeConversion  OutDataTypeStr=uint8  RndMeth=Round
  CAN5_ID4_message_ALTU : Outport
  wires:
  Data Type Conversion/1 -> CAN5_ID4_message_ALTU/1
  ID4messageALTU/1 -> Data Type Conversion/1

== system halout/HAL_OUT/CAN5/FD5_Debug1_0x4D0/IDinALTU ==
  IDinALTU : Inport
  Data Type Conversion : DataTypeConversion  OutDataTypeStr=uint32  RndMeth=Round
  CAN5_IDin_ALTU : Outport
  wires:
  Data Type Conversion/1 -> CAN5_IDin_ALTU/1
  IDinALTU/1 -> Data Type Conversion/1

== system halout/HAL_OUT/CAN5/FD5_Debug1_0x4D0/LFSensorMode ==
  LFSensorMode : Inport
  Data Type Conversion : DataTypeConversion  OutDataTypeStr=uint8  RndMeth=Round
  CAN5_LFSensorMode : Outport
  wires:
  Data Type Conversion/1 -> CAN5_LFSensorMode/1
  LFSensorMode/1 -> Data Type Conversion/1

== system halout/HAL_OUT/CAN5/FD5_Debug1_0x4D0/LRSensorMode ==
  LRSensorMode : Inport
  Data Type Conversion : DataTypeConversion  OutDataTypeStr=uint8  RndMeth=Round
  CAN5_LRSensorMode : Outport
  wires:
  Data Type Conversion/1 -> CAN5_LRSensorMode/1
  LRSensorMode/1 -> Data Type Conversion/1

== system halout/HAL_OUT/CAN5/FD5_Debug1_0x4D0/RFFATALTU ==
  RFFATALTU : Inport
  Data Type Conversion : DataTypeConversion  OutDataTypeStr=uint8  RndMeth=Round
  CAN5_RF_FAT_ALTU : Outport
  wires:
  Data Type Conversion/1 -> CAN5_RF_FAT_ALTU/1
  RFFATALTU/1 -> Data Type Conversion/1

== system halout/HAL_OUT/CAN5/FD5_Debug1_0x4D0/RFSensorMode ==
  RFSensorMode : Inport
  Data Type Conversion : DataTypeConversion  OutDataTypeStr=uint8  RndMeth=Round
  CAN5_RFSensorMode : Outport
  wires:
  Data Type Conversion/1 -> CAN5_RFSensorMode/1
  RFSensorMode/1 -> Data Type Conversion/1

== system halout/HAL_OUT/CAN5/FD5_Debug1_0x4D0/RRSensorMode ==
  RRSensorMode : Inport
  Data Type Conversion : DataTypeConversion  OutDataTypeStr=uint8  RndMeth=Round
  CAN5_RRSensorMode : Outport
  wires:
  Data Type Conversion/1 -> CAN5_RRSensorMode/1
  RRSensorMode/1 -> Data Type Conversion/1

== system halout/HAL_OUT/CAN5/FD5_Debug1_0x4D0/S1WheelDebugALTU ==
  S1WheelDebugALTU : Inport
  Data Type Conversion : DataTypeConversion  OutDataTypeStr=uint8  RndMeth=Round
  convert_out : FVT_lib/hal/convert_out  gain=0.5  offset=0
  CAN5_S1WheelDebug_ALTU : Outport
  wires:
  Data Type Conversion/1 -> CAN5_S1WheelDebug_ALTU/1
  convert_out/1 -> Data Type Conversion/1
  S1WheelDebugALTU/1 -> convert_out/1

== system halout/HAL_OUT/CAN5/FD5_Debug1_0x4D0/S2WheelDebugALTU ==
  S2WheelDebugALTU : Inport
  Data Type Conversion : DataTypeConversion  OutDataTypeStr=uint8  RndMeth=Round
  convert_out : FVT_lib/hal/convert_out  gain=0.5  offset=0
  CAN5_S2WheelDebug_ALTU : Outport
  wires:
  Data Type Conversion/1 -> CAN5_S2WheelDebug_ALTU/1
  convert_out/1 -> Data Type Conversion/1
  S2WheelDebugALTU/1 -> convert_out/1

== system halout/HAL_OUT/CAN5/FD5_Debug1_0x4D0/S3WheelDebugALTU ==
  S3WheelDebugALTU : Inport
  Data Type Conversion : DataTypeConversion  OutDataTypeStr=uint8  RndMeth=Round
  convert_out : FVT_lib/hal/convert_out  gain=0.5  offset=0
  CAN5_S3WheelDebug_ALTU : Outport
  wires:
  Data Type Conversion/1 -> CAN5_S3WheelDebug_ALTU/1
  convert_out/1 -> Data Type Conversion/1
  S3WheelDebugALTU/1 -> convert_out/1

== system halout/HAL_OUT/CAN5/FD5_Debug1_0x4D0/S4WheelDebugALTU ==
  S4WheelDebugALTU : Inport
  Data Type Conversion : DataTypeConversion  OutDataTypeStr=uint8  RndMeth=Round
  convert_out : FVT_lib/hal/convert_out  gain=0.5  offset=0
  CAN5_S4WheelDebug_ALTU : Outport
  wires:
  Data Type Conversion/1 -> CAN5_S4WheelDebug_ALTU/1
  convert_out/1 -> Data Type Conversion/1
  S4WheelDebugALTU/1 -> convert_out/1

== system halout/HAL_OUT/CAN5/FD5_Debug2_0x4F7/FDCDKCA0UWBEventSta ==
  FDCDKCA0UWBEventSta : Inport
  Data Type Conversion : DataTypeConversion  OutDataTypeStr=uint8  RndMeth=Round
  CAN5_FDC_DKC_A0_UWB_Event_Sta : Outport
  wires:
  Data Type Conversion/1 -> CAN5_FDC_DKC_A0_UWB_Event_Sta/1
  FDCDKCA0UWBEventSta/1 -> Data Type Conversion/1

== system halout/HAL_OUT/CAN5/FD5_Debug2_0x4F7/FDCDKCAllowSleepSta ==
  FDCDKCAllowSleepSta : Inport
  Data Type Conversion : DataTypeConversion  OutDataTypeStr=uint8  RndMeth=Round
  CAN5_FDC_DKC_AllowSleep_Sta : Outport
  wires:
  Data Type Conversion/1 -> CAN5_FDC_DKC_AllowSleep_Sta/1
  FDCDKCAllowSleepSta/1 -> Data Type Conversion/1

== system halout/HAL_OUT/CAN5/FD5_Debug2_0x4F7/FDCDKCBLERSSISta ==
  FDCDKCBLERSSISta : Inport
  Data Type Conversion : DataTypeConversion  OutDataTypeStr=uint8  RndMeth=Round
  CAN5_FDC_DKC_BLERSSI_Sta : Outport
  wires:
  Data Type Conversion/1 -> CAN5_FDC_DKC_BLERSSI_Sta/1
  FDCDKCBLERSSISta/1 -> Data Type Conversion/1

== system halout/HAL_OUT/CAN5/FD5_Debug2_0x4F7/FDCDKCBLEdcEventSta ==
  FDCDKCBLEdcEventSta : Inport
  Data Type Conversion : DataTypeConversion  OutDataTypeStr=uint8  RndMeth=Round
  CAN5_FDC_DKC_BLEdcEvent_Sta : Outport
  wires:
  Data Type Conversion/1 -> CAN5_FDC_DKC_BLEdcEvent_Sta/1
  FDCDKCBLEdcEventSta/1 -> Data Type Conversion/1

== system halout/HAL_OUT/CAN5/FD5_Debug2_0x4F7/FDCDKCCalDistanceSta ==
  FDCDKCCalDistanceSta : Inport
  Data Type Conversion : DataTypeConversion  OutDataTypeStr=uint8  RndMeth=Round
  CAN5_FDC_DKC_CalDistance_Sta : Outport
  wires:
  Data Type Conversion/1 -> CAN5_FDC_DKC_CalDistance_Sta/1
  FDCDKCCalDistanceSta/1 -> Data Type Conversion/1

== system halout/HAL_OUT/CAN5/FD5_Debug2_0x4F7/FDCDKCCommandToBCMCmd ==
  FDCDKCCommandToBCMCmd : Inport
  Data Type Conversion : DataTypeConversion  OutDataTypeStr=uint8  RndMeth=Round
  CAN5_FDC_DKC_CommandToBCM_Cmd : Outport
  wires:
  Data Type Conversion/1 -> CAN5_FDC_DKC_CommandToBCM_Cmd/1
  FDCDKCCommandToBCMCmd/1 -> Data Type Conversion/1

== system halout/HAL_OUT/CAN5/FD5_Debug2_0x4F7/FDCDKCCoordinateXSta ==
  FDCDKCCoordinateXSta : Inport
  Data Type Conversion : DataTypeConversion  OutDataTypeStr=uint16  RndMeth=Round
  convert_out : FVT_lib/hal/convert_out  gain=10  offset=-2550
  CAN5_FDC_DKC_CoordinateX_Sta : Outport
  wires:
  Data Type Conversion/1 -> CAN5_FDC_DKC_CoordinateX_Sta/1
  convert_out/1 -> Data Type Conversion/1
  FDCDKCCoordinateXSta/1 -> convert_out/1

== system halout/HAL_OUT/CAN5/FD5_Debug2_0x4F7/FDCDKCCoordinateYSta ==
  FDCDKCCoordinateYSta : Inport
  Data Type Conversion : DataTypeConversion  OutDataTypeStr=uint16  RndMeth=Round
  convert_out : FVT_lib/hal/convert_out  gain=10  offset=-2550
  CAN5_FDC_DKC_CoordinateY_Sta : Outport
  wires:
  Data Type Conversion/1 -> CAN5_FDC_DKC_CoordinateY_Sta/1
  convert_out/1 -> Data Type Conversion/1
  FDCDKCCoordinateYSta/1 -> convert_out/1

== system halout/HAL_OUT/CAN5/FD5_Debug2_0x4F7/FDCDKCDKeyAreaPESta ==
  FDCDKCDKeyAreaPESta : Inport
  Data Type Conversion : DataTypeConversion  OutDataTypeStr=uint8  RndMeth=Round
  CAN5_FDC_DKC_DKeyAreaPE_Sta : Outport
  wires:
  Data Type Conversion/1 -> CAN5_FDC_DKC_DKeyAreaPE_Sta/1
  FDCDKCDKeyAreaPESta/1 -> Data Type Conversion/1

== system halout/HAL_OUT/CAN5/FD5_Debug2_0x4F7/FDCDKCDKeyAreaPSSta ==
  FDCDKCDKeyAreaPSSta : Inport
  Data Type Conversion : DataTypeConversion  OutDataTypeStr=uint8  RndMeth=Round
  CAN5_FDC_DKC_DKeyAreaPS_Sta : Outport
  wires:
  Data Type Conversion/1 -> CAN5_FDC_DKC_DKeyAreaPS_Sta/1
  FDCDKCDKeyAreaPSSta/1 -> Data Type Conversion/1

== system halout/HAL_OUT/CAN5/FD5_Debug2_0x4F7/FDCDKCDKeyAreaPTGSta ==
  FDCDKCDKeyAreaPTGSta : Inport
  Data Type Conversion : DataTypeConversion  OutDataTypeStr=uint8  RndMeth=Round
  CAN5_FDC_DKC_DKeyAreaPTG_Sta : Outport
  wires:
  Data Type Conversion/1 -> CAN5_FDC_DKC_DKeyAreaPTG_Sta/1
  FDCDKCDKeyAreaPTGSta/1 -> Data Type Conversion/1

== system halout/HAL_OUT/CAN5/FD5_Debug2_0x4F7/FDCDKCDKeyAreaSPTGSta ==
  FDCDKCDKeyAreaSPTGSta : Inport
  Data Type Conversion : DataTypeConversion  OutDataTypeStr=uint8  RndMeth=Round
  CAN5_FDC_DKC_DKeyAreaSPTG_Sta : Outport
  wires:
  Data Type Conversion/1 -> CAN5_FDC_DKC_DKeyAreaSPTG_Sta/1
  FDCDKCDKeyAreaSPTGSta/1 -> Data Type Conversion/1

== system halout/HAL_OUT/CAN5/FD5_Debug2_0x4F7/FDCDKCDKeyWelcomeSta ==
  FDCDKCDKeyWelcomeSta : Inport
  Data Type Conversion : DataTypeConversion  OutDataTypeStr=uint8  RndMeth=Round
  CAN5_FDC_DKC_DKeyWelcome_Sta : Outport
  wires:
  Data Type Conversion/1 -> CAN5_FDC_DKC_DKeyWelcome_Sta/1
  FDCDKCDKeyWelcomeSta/1 -> Data Type Conversion/1

== system halout/HAL_OUT/CAN5/FD5_Debug2_0x4F7/FDCDKCDkeyAreaRAPSSta ==
  FDCDKCDkeyAreaRAPSSta : Inport
  Data Type Conversion : DataTypeConversion  OutDataTypeStr=uint8  RndMeth=Round
  CAN5_FDC_DKC_DkeyAreaRAPS_Sta : Outport
  wires:
  Data Type Conversion/1 -> CAN5_FDC_DKC_DkeyAreaRAPS_Sta/1
  FDCDKCDkeyAreaRAPSSta/1 -> Data Type Conversion/1

== system halout/HAL_OUT/CAN5/FD5_Debug2_0x4F7/FDCDKCDkeyShowIVISta ==
  FDCDKCDkeyShowIVISta : Inport
  Data Type Conversion : DataTypeConversion  OutDataTypeStr=uint8  RndMeth=Round
  CAN5_FDC_DKC_DkeyShowIVI_Sta : Outport
  wires:
  Data Type Conversion/1 -> CAN5_FDC_DKC_DkeyShowIVI_Sta/1
  FDCDKCDkeyShowIVISta/1 -> Data Type Conversion/1

== system halout/HAL_OUT/CAN5/FD5_Debug2_0x4F7/FDCDKCKeyMissSta ==
  FDCDKCKeyMissSta : Inport
  Data Type Conversion : DataTypeConversion  OutDataTypeStr=uint8  RndMeth=Round
  CAN5_FDC_DKC_KeyMiss_Sta : Outport
  wires:
  Data Type Conversion/1 -> CAN5_FDC_DKC_KeyMiss_Sta/1
  FDCDKCKeyMissSta/1 -> Data Type Conversion/1

== system halout/HAL_OUT/CAN5/FD5_Debug2_0x4F7/FDCDKCKeyModeSta ==
  FDCDKCKeyModeSta : Inport
  Data Type Conversion : DataTypeConversion  OutDataTypeStr=uint8  RndMeth=Round
  CAN5_FDC_DKC_KeyMode_Sta : Outport
  wires:
  Data Type Conversion/1 -> CAN5_FDC_DKC_KeyMode_Sta/1
  FDCDKCKeyModeSta/1 -> Data Type Conversion/1

== system halout/HAL_OUT/CAN5/FD5_Debug2_0x4F7/FDCDKCKeyNumSta ==
  FDCDKCKeyNumSta : Inport
  Data Type Conversion : DataTypeConversion  OutDataTypeStr=uint8  RndMeth=Round
  CAN5_FDC_DKC_KeyNum_Sta : Outport
  wires:
  Data Type Conversion/1 -> CAN5_FDC_DKC_KeyNum_Sta/1
  FDCDKCKeyNumSta/1 -> Data Type Conversion/1

== system halout/HAL_OUT/CAN5/FD5_Debug2_0x4F7/FDCDKCKeyTypeSta ==
  FDCDKCKeyTypeSta : Inport
  Data Type Conversion : DataTypeConversion  OutDataTypeStr=uint8  RndMeth=Round
  CAN5_FDC_DKC_KeyType_Sta : Outport
  wires:
  Data Type Conversion/1 -> CAN5_FDC_DKC_KeyType_Sta/1
  FDCDKCKeyTypeSta/1 -> Data Type Conversion/1

== system halout/HAL_OUT/CAN5/FD5_Debug2_0x4F7/FDCDKCOutputPCMDModuleSta ==
  FDCDKCOutputPCMDModuleSta : Inport
  Data Type Conversion : DataTypeConversion  OutDataTypeStr=uint8  RndMeth=Round
  CAN5_FDC_DKC_OutputPCMDModule_Sta : Outport
  wires:
  Data Type Conversion/1 -> CAN5_FDC_DKC_OutputPCMDModule_Sta/1
  FDCDKCOutputPCMDModuleSta/1 -> Data Type Conversion/1

== system halout/HAL_OUT/CAN5/FD5_Debug2_0x4F7/FDCDKCParkingModeCmd ==
  FDCDKCParkingModeCmd : Inport
  Data Type Conversion : DataTypeConversion  OutDataTypeStr=uint8  RndMeth=Round
  CAN5_FDC_DKC_ParkingMode_Cmd : Outport
  wires:
  Data Type Conversion/1 -> CAN5_FDC_DKC_ParkingMode_Cmd/1
  FDCDKCParkingModeCmd/1 -> Data Type Conversion/1

== system halout/HAL_OUT/CAN5/FD5_Debug2_0x4F7/FDCDKCReVehDataSta ==
  FDCDKCReVehDataSta : Inport
  Data Type Conversion : DataTypeConversion  OutDataTypeStr=uint8  RndMeth=Round
  CAN5_FDC_DKC_ReVehData_Sta : Outport
  wires:
  Data Type Conversion/1 -> CAN5_FDC_DKC_ReVehData_Sta/1
  FDCDKCReVehDataSta/1 -> Data Type Conversion/1

== system halout/HAL_OUT/CAN5/FD5_Debug2_0x4F7/FDCDKCRemoLeftPSDCmd ==
  FDCDKCRemoLeftPSDCmd : Inport
  Data Type Conversion : DataTypeConversion  OutDataTypeStr=uint8  RndMeth=Round
  CAN5_FDC_DKC_RemoLeftPSD_Cmd : Outport
  wires:
  Data Type Conversion/1 -> CAN5_FDC_DKC_RemoLeftPSD_Cmd/1
  FDCDKCRemoLeftPSDCmd/1 -> Data Type Conversion/1
